simulink model "obs_com_filtro_2014"  (R2014b)
settings: Solver=ode45  SolverMode=SingleTasking  StartTime=0.0  StopTime=600  RelTol=1e-3
model workspace (MAT data in the model file):
  Td = 2
  std_dev = 0.08
values from neighbouring files (symbols this model uses):
  K = 0.002677    [run_and_calculate.m]
  T = 0.5    [run_and_calculate.m]
undefined symbols (not defined in the file): sigma_n
libraries: cstblocks x27
(part 1 of 2)
settings Model: CovMetricSettings=dwe  CovHtmlReporting=off  covSaveCumulativeToWorkspaceVar=off  CovSaveSingleToWorkspaceVar=off  CovExternalEMLEnable=on  CovSFcnEnable=on  Creator=Gabriel Vieira  LastModifiedBy=Gabriel Vieira
settings DataIOCC: LimitDataPoints=off  SaveFormat=StructureWithTime  ReturnWorkspaceOutputs=on
settings DebuggingCC: SolverPrmCheckMsg=none  FrameProcessingCompatibilityMsg=error  SFUnexpectedBacktrackingDiag=error  SFNoUnconditionalDefaultTransitionDiag=error
settings HardwareCC: ProdBitPerPointer=64  ProdLargestAtomicFloat=Float  ProdIntDivRoundTo=Zero  ProdEndianess=LittleEndian  ProdHWDeviceType=Specified
settings ModelReferenceCC: PropagateSignalLabelsOutOfModel=on
settings SFSimCC: SimUseLocalCustomCode=on
settings RTWCC: RTWUseLocalCustomCode=on
settings GRTTargetCC: TargetLangStandard=C99 (ISO)

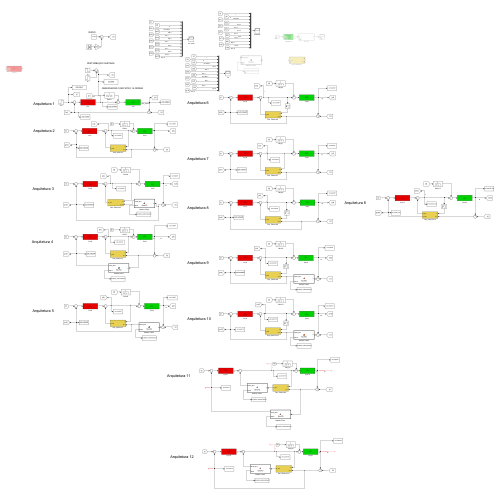
[thumbnail: Simulink's stored preview of the top-level diagram]
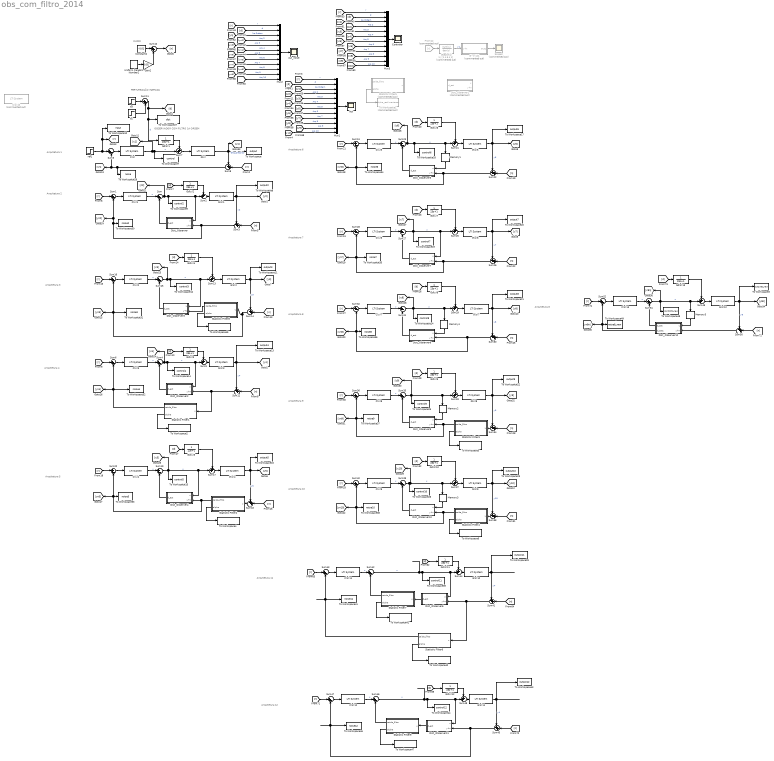
== system obs_com_filtro_2014 ==
  note: RUÍDO
  note: OBSERVADOR COM FILTRO 1A ORDEM
  note: PERTURBAÇÃO INJETADA
  note: Arquitetura 1
  note: Arquitetura 2
  note: Arquitetura 3
  note: Arquitetura 4
  note: Arquitetura 5
  note: Arquitetura 6
  note: Arquitetura 7
  note: Arquitetura 8
  note: Arquitetura 9
  note: Arquitetura 10
  note: Arquitetura 11
  note: Arquitetura 12
  note: Arquitetura 8
  C(s){,1..9,11..13} (13 alike) : cstblocks/LTI System  sys=C  IC=[]
  C(s)10 : cstblocks/LTI System  Commented=on  sys=C  IC=[]
  Constant2 : Constant  Value=-0.01
  Controler : Scope
      settings: TimeRange=auto  ShowLegends=on  MaxDataPoints=5000  SaveToWorkspace=off  YMin=-31.53639  YMax=49.84802  SampleTime=-1
  Dist_Observer : Subsystem  mask{Td=Td}
      mask prompts: Td "Filter time cte (Td)"
  Dist_Observer1 : Subsystem  Commented=on  mask{std_dev=std_dev}
      mask prompts: std_dev "Noise Std Deviation (std_dev)"
  Dist_Observer10 : Subsystem  mask{Td=Td, std_dev=std_dev}
      mask prompts: Td "Filter time cte (Td)"; std_dev "Noised Std Derivation"
  Dist_Observer11 : Subsystem  mask{Td=Td}
      mask prompts: Td "Filter time cte (Td)"
  Dist_Observer12 : Subsystem  mask{std_dev=std_dev}
      mask prompts: std_dev "Noised Std Derivation"
  Dist_Observer2 : Subsystem  mask{Td=Td}
      mask prompts: Td "Filter time cte (Td)"
  Dist_Observer3 : Subsystem  mask{Td=Td}
      mask prompts: Td "Filter time cte (Td)"
  Dist_Observer4 : Subsystem  mask{Td=Td}
      mask prompts: Td "Filter time cte (Td)"
  Dist_Observer5 : Subsystem  mask{Td=Td, std_dev=std_dev}
      mask prompts: Td "Filter time cte (Td)"; std_dev "Noised Std Derivation"
  Dist_Observer6 : Subsystem  mask{Td=Td}
      mask prompts: Td "Filter time cte (Td)"
  Dist_Observer7 : Subsystem  mask{Td=Td, std_dev=std_dev}
      mask prompts: Td "Filter time cte (Td)"; std_dev "Noised Std Derivation"
  Dist_Observer8 : Subsystem  mask{std_dev=std_dev}
      mask prompts: std_dev "Noised Std Derivation"
  Dist_Observer9 : Subsystem  mask{Td=Td, std_dev=std_dev}
      mask prompts: Td "Filter time cte (Td)"; std_dev "Noised Std Derivation"
  From12 : From  Commented=on  GotoTag=r
  G(s){,1..12} (13 alike) : cstblocks/LTI System  sys=Gs  IC=[]
  "G^{-1}1" : Subsystem  Commented=on
  Gain2 : Gain  Gain=0.02
  Gd(s){1..13} (13 alike) : TransferFcn  Numerator=1  Denominator=[23 1]
  Gteste(s) : TransferFcn  Commented=on  Numerator=1  Denominator=[1 4 6 4 1]
  Memory{1..5} (5 alike) : Memory
  Mux1 : Mux  Inputs=12
  Mux2 : Mux  Inputs=12
  Mux3 : Mux  Inputs=12
  Scope2 : Scope  Commented=on
  Statistic Filter1 : MATLAB Function  TreatAsAtomicUnit=on  mask{std_dev=sigma_n}
      mask prompts: std_dev "Noise Std Deviation (std_dev)"
      settings: PermitHierarchicalResolution=ParametersOnly
  Statistic Filter2 : MATLAB Function  TreatAsAtomicUnit=on  mask{std_dev=sigma_n}
      mask prompts: std_dev "Noise Std Deviation (std_dev)"
      settings: PermitHierarchicalResolution=ParametersOnly
  Statistic Filter3 : MATLAB Function  TreatAsAtomicUnit=on  mask{std_dev=sigma_n}
      mask prompts: std_dev "Noise Std Deviation (std_dev)"
      settings: PermitHierarchicalResolution=ParametersOnly
  Statistic Filter4 : MATLAB Function  TreatAsAtomicUnit=on  mask{std_dev=sigma_n}
      mask prompts: std_dev "Noise Std Deviation (std_dev)"
      settings: PermitHierarchicalResolution=ParametersOnly
  Statistic Filter5 : MATLAB Function  Commented=on  TreatAsAtomicUnit=on  mask{std_dev=0.5}
      mask prompts: std_dev "Noise Std Deviation (std_dev)"
      settings: PermitHierarchicalResolution=ParametersOnly
  Statistic Filter6 : MATLAB Function  TreatAsAtomicUnit=on  mask{std_dev=sigma_n}
      mask prompts: std_dev "Noise Std Deviation (std_dev)"
      settings: PermitHierarchicalResolution=ParametersOnly
  Statistic Filter7 : MATLAB Function  TreatAsAtomicUnit=on  mask{std_dev=sigma_n*2}
      mask prompts: std_dev "Noise Std Deviation (std_dev)"
      settings: PermitHierarchicalResolution=ParametersOnly
  Statistic Filter8 : MATLAB Function  TreatAsAtomicUnit=on  mask{std_dev=sigma_n}
      mask prompts: std_dev "Noise Std Deviation (std_dev)"
      settings: PermitHierarchicalResolution=ParametersOnly
  Statistic Filter9 : MATLAB Function  TreatAsAtomicUnit=on  mask{std_dev=sigma_n}
      mask prompts: std_dev "Noise Std Deviation (std_dev)"
      settings: PermitHierarchicalResolution=ParametersOnly
  Sum{,1,4..6,15..16,19..20,23..24,27..28,31..32,35..36,39..40,42..43,46..47,51..52} (25 alike) : Sum  Inputs=|+-
  Sum10 : Sum  Inputs=|++
  Sum11 : Sum  Inputs=|++
  Sum{2..3,7..9,12..14,17..18,21..22,25..26,29..30,33..34,37..38,41,44..45,48..50} (26 alike) : Sum  Inputs=++|
  To Workspace : ToWorkspace  VariableName=output  SaveFormat=Timeseries  SampleTime=-1
  To Workspace1 : ToWorkspace  Commented=on  VariableName=alpha_realimentacao  SaveFormat=Timeseries  SampleTime=-1
  To Workspace10 : ToWorkspace  VariableName=input  SaveFormat=Timeseries  SampleTime=-1
  To Workspace11 : ToWorkspace  VariableName=output3  SaveFormat=Timeseries  SampleTime=-1
  To Workspace12 : ToWorkspace  VariableName=control3  SaveFormat=Timeseries  SampleTime=-1
  To Workspace13 : ToWorkspace  VariableName=output4  SaveFormat=Timeseries  SampleTime=-1
  To Workspace14 : ToWorkspace  VariableName=control4  SaveFormat=Timeseries  SampleTime=-1
  To Workspace15 : ToWorkspace  VariableName=control5  SaveFormat=Timeseries  SampleTime=-1
  To Workspace16 : ToWorkspace  VariableName=output5  SaveFormat=Timeseries  SampleTime=-1
  To Workspace17 : ToWorkspace  VariableName=output6  SaveFormat=Timeseries  SampleTime=-1
  To Workspace18 : ToWorkspace  VariableName=control6  SaveFormat=Timeseries  SampleTime=-1
  To Workspace19 : ToWorkspace  VariableName=control7  SaveFormat=Timeseries  SampleTime=-1
  To Workspace2 : ToWorkspace  VariableName=alpha_realimentacao1  SaveFormat=Timeseries  SampleTime=-1
  To Workspace20 : ToWorkspace  VariableName=output7  SaveFormat=Timeseries  SampleTime=-1
  To Workspace21 : ToWorkspace  VariableName=output8  SaveFormat=Timeseries  SampleTime=-1
  To Workspace22 : ToWorkspace  VariableName=output9  SaveFormat=Timeseries  SampleTime=-1
  To Workspace23 : ToWorkspace  VariableName=output10  SaveFormat=Timeseries  SampleTime=-1
  To Workspace24 : ToWorkspace  VariableName=control8  SaveFormat=Timeseries  SampleTime=-1
  To Workspace25 : ToWorkspace  VariableName=control9  SaveFormat=Timeseries  SampleTime=-1
  To Workspace26 : ToWorkspace  VariableName=control10  SaveFormat=Timeseries  SampleTime=-1
  To Workspace27 : ToWorkspace  VariableName=dist  SaveFormat=Timeseries  SampleTime=-1
  To Workspace28 : ToWorkspace  VariableName=noise  SaveFormat=Timeseries  SampleTime=-1
  To Workspace29 : ToWorkspace  VariableName=output11  SaveFormat=Timeseries  SampleTime=-1
  To Workspace3 : ToWorkspace  VariableName=output8_new  SaveFormat=Timeseries  SampleTime=-1
  To Workspace30 : ToWorkspace  VariableName=noise2  SaveFormat=Timeseries  SampleTime=-1
  To Workspace31 : ToWorkspace  VariableName=noise3  SaveFormat=Timeseries  SampleTime=-1
  To Workspace32 : ToWorkspace  VariableName=noise4  SaveFormat=Timeseries  SampleTime=-1
  To Workspace33 : ToWorkspace  VariableName=noise5  SaveFormat=Timeseries  SampleTime=-1
  To Workspace34 : ToWorkspace  VariableName=noise6  SaveFormat=Timeseries  SampleTime=-1
  To Workspace35 : ToWorkspace  VariableName=noise7  SaveFormat=Timeseries  SampleTime=-1
  To Workspace36 : ToWorkspace  VariableName=noise8  SaveFormat=Timeseries  SampleTime=-1
  To Workspace37 : ToWorkspace  VariableName=noise9  SaveFormat=Timeseries  SampleTime=-1
  To Workspace38 : ToWorkspace  VariableName=noise10  SaveFormat=Timeseries  SampleTime=-1
  To Workspace39 : ToWorkspace  VariableName=control11  SaveFormat=Timeseries  SampleTime=-1
  To Workspace4 : ToWorkspace  VariableName=alpha_realimentacao3  SaveFormat=Timeseries  SampleTime=-1
  To Workspace40 : ToWorkspace  VariableName=alpha_realimentacao11  SaveFormat=Timeseries  SampleTime=-1
  To Workspace41 : ToWorkspace  VariableName=noise11  SaveFormat=Timeseries  SampleTime=-1
  To Workspace42 : ToWorkspace  VariableName=alpha_realimentacao8  SaveFormat=Timeseries  SampleTime=-1
  To Workspace43 : ToWorkspace  VariableName=output12  SaveFormat=Timeseries  SampleTime=-1
  To Workspace44 : ToWorkspace  VariableName=control12  SaveFormat=Timeseries  SampleTime=-1
  To Workspace45 : ToWorkspace  VariableName=alpha_realimentacao9  SaveFormat=Timeseries  SampleTime=-1
  To Workspace46 : ToWorkspace  VariableName=noise12  SaveFormat=Timeseries  SampleTime=-1
  To Workspace47 : ToWorkspace  VariableName=alpha_realimentacao12  SaveFormat=Timeseries  SampleTime=-1
  To Workspace48 : ToWorkspace  VariableName=control8_new  SaveFormat=Timeseries  SampleTime=-1
  To Workspace49 : ToWorkspace  VariableName=noise8_new  SaveFormat=Timeseries  SampleTime=-1
  To Workspace5 : ToWorkspace  VariableName=alpha_realimentacao4  SaveFormat=Timeseries  SampleTime=-1
  To Workspace6 : ToWorkspace  VariableName=alpha_realimentacao6  SaveFormat=Timeseries  SampleTime=-1
  To Workspace7 : ToWorkspace  VariableName=control  SaveFormat=Timeseries  SampleTime=-1
  To Workspace8 : ToWorkspace  VariableName=output2  SaveFormat=Timeseries  SampleTime=-1
  To Workspace9 : ToWorkspace  VariableName=control2  SaveFormat=Timeseries  SampleTime=-1
  Uniform Random Number2 : UniformRandomNumber  SampleTime=0.01
  d2 : Step  Time=150  SampleTime=0
  d3 : Step  Time=200  After=-1  SampleTime=0
  out : Scope
  out_noise : Scope
  ref1 : Step  Time=50  SampleTime=0
  wires:
  Sum10/1 -> [n]
  Constant2/1 -> Sum10/1
  Sum5/1 -> C(s)/1
  d2/1 -> Sum11/2
  C(s)/1 -> [c1], To Workspace7/1, Sum7/2  "u"
  Gain2/1 -> Sum10/2
  ref1/1 -> To Workspace10/1, [r], Sum5/1
  Uniform Random Number2/1 -> Gain2/1
  Mux1/1 -> out/1
  Sum7/1 -> G(s)/1
  Sum11/1 -> [d], To Workspace27/1, Gd(s)1/1  "d"
  Gd(s)1/1 -> Sum7/1
  [n] -> Sum8/2
  d3/1 -> Sum11/1
  G(s)/1 -> [y1], Sum8/1, To Workspace/1  "Obs_Classico"
  Sum8/1 -> To Workspace28/1, [yn], Sum5/2
  [n] -> Sum3/2
  Gd(s)2/1 -> Sum2/1
  Sum2/1 -> G(s)1/1
  Sum1/1 -> C(s)1/1
  [r] -> Sum1/1
  [d] -> Gd(s)2/1
  C(s)1/1 -> Sum/1  "u"
  Sum3/1 -> Dist_Observer/2(y+n), To Workspace30/1, [yn2], Sum1/2
  Dist_Observer/1(d_est) -> Sum/2
  G(s)1/1 -> To Workspace8/1, [y2], Sum3/1  "y2"
  Statistic Filter5/2(alpha) -> To Workspace1/1
  Sum9/1 -> G(s)3/1
  Gd(s)3/1 -> Sum9/1
  G(s)3/1 -> To Workspace13/1, [y4], Sum12/1  "y4"
  [r] -> Sum6/1
  [d] -> Gd(s)3/1
  C(s)3/1 -> Sum4/1  "u"
  Dist_Observer2/1(d_est) -> Sum4/2
  Sum6/1 -> C(s)3/1
  [n] -> Sum12/2
  Sum12/1 -> Statistic Filter1/1(u), Dist_Observer2/2(y+n)
  Statistic Filter1/2(alpha) -> To Workspace2/1
  Gteste(s)/1 -> "G^{-1}1"/1(y+n)  "y1"
  From12/1 -> Gteste(s)/1
  "G^{-1}1"/1(Out1) -> Scope2/1
  [d] -> Gd(s)4/1
  Sum13/1 -> G(s)2/1
  Gd(s)4/1 -> Sum13/1
  [n] -> Sum14/2
  G(s)2/1 -> Sum14/1, To Workspace11/1, [y3]  "y3"
  Sum16/1 -> C(s)2/1
  C(s)2/1 -> Sum15/1  "u"
  [r] -> Sum16/1
  Dist_Observer4/1(d_est) -> Sum19/2
  [r] -> Sum20/1
  Sum17/1 -> G(s)4/1
  Sum18/1 -> Statistic Filter2/1(u)
  Statistic Filter2/2(alpha) -> To Workspace4/1
  G(s)4/1 -> To Workspace16/1, [y5], Sum18/1  "y5"
  [d] -> Gd(s)5/1
  Sum20/1 -> C(s)4/1
  C(s)4/1 -> Sum19/1  "u"
  Gd(s)5/1 -> Sum17/1
  [n] -> Sum18/2
  [n] -> Sum22/2
  Gd(s)6/1 -> Sum21/1
  Sum24/1 -> C(s)5/1
  [d] -> Gd(s)6/1
  C(s)5/1 -> Sum23/1  "u"
  G(s)5/1 -> To Workspace17/1, [y6], Sum22/1  "y6"
  Dist_Observer5/1(d_est) -> Sum23/2
  Sum21/1 -> G(s)5/1
  [r] -> Sum24/1
  Gd(s)7/1 -> Sum25/1
  [n] -> Sum26/2
  G(s)6/1 -> To Workspace20/1, [y7], Sum26/1  "y7"
  Sum28/1 -> C(s)6/1
  C(s)6/1 -> Sum27/1  "u"
  [r] -> Sum28/1
  Dist_Observer7/1(d_est) -> Sum27/2
  [d] -> Gd(s)7/1
  Sum25/1 -> G(s)6/1
  Gd(s)8/1 -> Sum29/1
  Dist_Observer8/1(d_est) -> Sum31/2
  [r] -> Sum32/1
  C(s)7/1 -> Sum31/1  "u"
  Sum32/1 -> C(s)7/1
  [n] -> Sum30/2
  G(s)7/1 -> To Workspace21/1, [y8], Sum30/1  "y8"
  Sum29/1 -> G(s)7/1
  Sum38/1 -> Statistic Filter4/1(u)
  Statistic Filter4/2(alpha) -> To Workspace6/1
  Gd(s)10/1 -> Sum37/1
  Dist_Observer10/1(d_est) -> Sum39/2
  G(s)9/1 -> To Workspace23/1, [y10], Sum38/1  "y10"
  [n] -> Sum38/2
  Sum34/1 -> Statistic Filter3/1(u)
  Sum40/1 -> C(s)9/1
  C(s)9/1 -> Sum39/1  "u"
  Statistic Filter3/2(alpha) -> To Workspace5/1
  Gd(s)9/1 -> Sum33/1
  Sum35/1 -> [c9], To Workspace25/1, Memory2/1, Sum33/2
  [n] -> Sum34/2
  G(s)8/1 -> [y9], To Workspace22/1, Sum34/1  "y9"
  [r] -> Sum36/1
  [r] -> Sum40/1
  Dist_Observer9/1(d_est) -> Sum35/2
  [d] -> Gd(s)9/1
  Sum33/1 -> G(s)8/1
  Sum37/1 -> G(s)9/1
  Sum36/1 -> C(s)8/1
  C(s)8/1 -> Sum35/1  "u"
  [d] -> Gd(s)10/1
  [r] -> Mux2/1  "r"
  [d] -> Mux2/2  "d"
  Mux2/1 -> out_noise/1
  [yn] -> Mux2/3  "1a Ordem"
  Sum14/1 -> Statistic Filter8/1(u), To Workspace31/1, [yn3], Sum16/2
  Statistic Filter1/1(saida_filtro) -> Sum6/2, To Workspace32/1, [yn4]
  Statistic Filter2/1(saida_filtro) -> Dist_Observer4/2(y+n), To Workspace33/1, [yn5], Sum20/2
  Sum22/1 -> Dist_Observer5/2(y+n), To Workspace34/1, [yn6], Sum24/2
  Sum26/1 -> Dist_Observer7/2(y+n), To Workspace35/1, [yn7], Sum28/2
  Statistic Filter3/1(saida_filtro) -> Dist_Observer9/2(y+n), To Workspace37/1, [yn9], Sum36/2
  Statistic Filter4/1(saida_filtro) -> Dist_Observer10/2(y+n), To Workspace38/1, [yn10], Sum40/2
  Memory2/1 -> Dist_Observer9/1(u)
  Memory3/1 -> Dist_Observer10/1(u)
  [yn8] -> Mux2/10  "Arq 8"
  [yn7] -> Mux2/9  "Arq 7"
  [yn6] -> Mux2/8  "Arq 6"
  [yn5] -> Mux2/7  "Arq 5"
  [yn4] -> Mux2/6  "Arq 4"
  [yn3] -> Mux2/5  "Arq 3"
  [yn2] -> Mux2/4  "Arq 2"
  Mux3/1 -> Controler/1
  Sum15/1 -> [c3], To Workspace12/1, Dist_Observer3/1(u), Sum13/2  "u"
  Sum4/1 -> [c4], To Workspace14/1, Dist_Observer2/1(u), Sum9/2  "u"
  Sum19/1 -> [c5], To Workspace15/1, Dist_Observer4/1(u), Sum17/2  "u"
  Sum23/1 -> [c6], To Workspace18/1, Memory1/1, Sum21/2  "u"
  Sum27/1 -> [c7], To Workspace19/1, Dist_Observer7/1(u), Sum25/2  "u"
  Sum31/1 -> [c8], Memory4/1, Sum29/2, To Workspace24/1  "u"
  Sum39/1 -> To Workspace26/1, [c10], Memory3/1, Sum37/2  "u"
  [r] -> Mux3/1  "r"
  [d] -> Mux3/2  "d"
  Sum/1 -> [c2], To Workspace9/1, Dist_Observer/1(u), Sum2/2
  Statistic Filter8/1(saida_filtro) -> Dist_Observer3/2(y+n)
  Dist_Observer3/1(d_est) -> Sum15/2
  [y2] -> Mux1/4  "Arq 2"
  [y7] -> Mux1/9  "Arq 7"
  [y6] -> Mux1/8  "Arq 6"
  [y4] -> Mux1/6  "Arq 4"
  [y8] -> Mux1/10  "Arq 8"
  [y3] -> Mux1/5  "Arq 3"
  [y1] -> Mux1/3  "1a Ordem"
  [d] -> Mux1/2  "d"
  [r] -> Mux1/1  "r"
  [y5] -> Mux1/7  "Arq 5"
  [c2] -> Mux3/4  "Arq 2"
  [c5] -> Mux3/7  "Arq 5"
  [c7] -> Mux3/9  "Arq 7"
  [c6] -> Mux3/8  "Arq 6"
  [c4] -> Mux3/6  "Arq 4"
  [c8] -> Mux3/10  "Arq 8"
  [c1] -> Mux3/3  "1a Ordem"
  [c3] -> Mux3/5  "Arq 3"
  [yn10] -> Mux2/12  "Arq 10"
  [c10] -> Mux3/12  "Arq 10"
  [y10] -> Mux1/12  "Arq 10"
  [yn9] -> Mux2/11  "Arq 9"
  [c9] -> Mux3/11  "Arq 9"
  [y9] -> Mux1/11  "Arq 9"
  [d] -> Gd(s)8/1
  Statistic Filter6/1(saida_filtro) -> Sum43/2, To Workspace41/1
  Sum42/1 -> To Workspace39/1, Dist_Observer6/1(u), Sum44/2  "u"
  Gd(s)11/1 -> Sum44/1
  Sum41/1 -> Statistic Filter6/1(u), Dist_Observer6/2(y+n)
  Sum44/1 -> G(s)10/1
  G(s)10/1 -> To Workspace29/1, Sum41/1  "y4"
  [d] -> Gd(s)11/1
  C(s)11/1 -> Sum42/1  "u"
  [n] -> Sum41/2
  Sum43/1 -> C(s)11/1
  Statistic Filter6/2(alpha) -> To Workspace40/1
  [r] -> Sum43/1
  Dist_Observer6/1(d_est) -> Statistic Filter7/1(u)
  Statistic Filter7/2(alpha) -> To Workspace42/1
  Statistic Filter7/1(saida_filtro) -> Sum42/2
  Dist_Observer11/1(d_est) -> Statistic Filter9/1(u)
  Statistic Filter9/2(alpha) -> To Workspace47/1
  Sum47/1 -> C(s)12/1
  [n] -> Sum45/2
  [r] -> Sum47/1
  [d] -> Gd(s)12/1
  C(s)12/1 -> Sum46/1  "u"
  Sum48/1 -> G(s)11/1
  G(s)11/1 -> To Workspace43/1, Sum45/1  "y4"
  Gd(s)12/1 -> Sum48/1
  Sum45/1 -> To Workspace46/1, Sum47/2, Dist_Observer11/2(y+n)
  Sum46/1 -> To Workspace44/1, Dist_Observer11/1(u), Sum48/2  "u"
  Statistic Filter9/1(saida_filtro) -> Sum46/2
  Statistic Filter8/2(alpha) -> To Workspace45/1
  Sum30/1 -> Sum32/2, [yn8], To Workspace36/1, Dist_Observer8/2(y+n)
  Dist_Observer12/2(d_est1) -> [yn8n], To Workspace49/1, Sum52/2
  [r] -> Sum52/1
  Dist_Observer12/1(d_est) -> Sum51/2
  [d] -> Gd(s)13/1
  Sum52/1 -> C(s)13/1
  Sum50/1 -> Dist_Observer12/2(y+n)
  Sum49/1 -> G(s)12/1
  G(s)12/1 -> To Workspace3/1, [y8n], Sum50/1  "y8"
  Sum51/1 -> [c8n], Memory5/1, Sum49/2, To Workspace48/1  "u"
  [n] -> Sum50/2
  C(s)13/1 -> Sum51/1  "u"
  Gd(s)13/1 -> Sum49/1
  Memory1/1 -> Dist_Observer5/1(u)
  Memory4/1 -> Dist_Observer8/1(u)
  Memory5/1 -> Dist_Observer12/1(u)

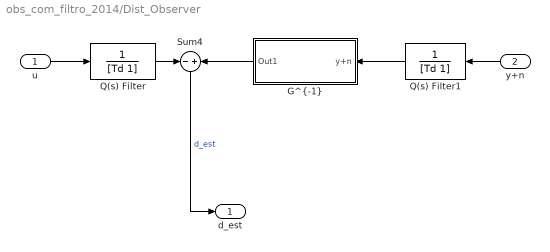
== system obs_com_filtro_2014/Dist_Observer ==
  u : Inport
  y+n : Inport  Port=2
  "G^{-1}" : Subsystem
  Q(s) Filter : TransferFcn  Denominator=[Td 1]
  Q(s) Filter1 : TransferFcn  Denominator=[Td 1]
  Sum4 : Sum  Inputs=-|+
  d_est : Outport
  wires:
  Q(s) Filter/1 -> Sum4/1
  Sum4/1 -> d_est/1  "d_est"
  u/1 -> Q(s) Filter/1
  "G^{-1}"/1(Out1) -> Sum4/2
  Q(s) Filter1/1 -> "G^{-1}"/1(y+n)
  y+n/1 -> Q(s) Filter1/1

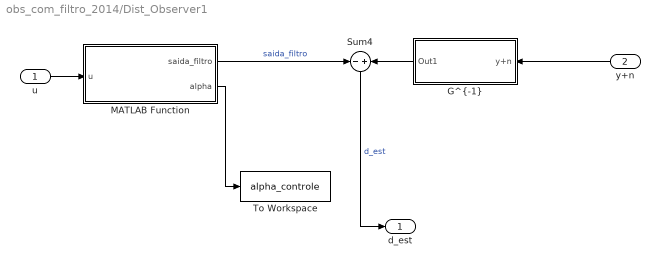
== system obs_com_filtro_2014/Dist_Observer1 ==
  u : Inport
  y+n : Inport  Port=2
  "G^{-1}" : Subsystem
  MATLAB Function : MATLAB Function  TreatAsAtomicUnit=on
      settings: PermitHierarchicalResolution=ParametersOnly
  Sum4 : Sum  Inputs=-|+
  To Workspace : ToWorkspace  VariableName=alpha_controle  SaveFormat=Timeseries  SampleTime=-1
  d_est : Outport
  wires:
  MATLAB Function/1(saida_filtro) -> Sum4/1  "saida_filtro"
  Sum4/1 -> d_est/1  "d_est"
  u/1 -> MATLAB Function/1(u)
  "G^{-1}"/1(Out1) -> Sum4/2
  MATLAB Function/2(alpha) -> To Workspace/1
  y+n/1 -> "G^{-1}"/1(y+n)

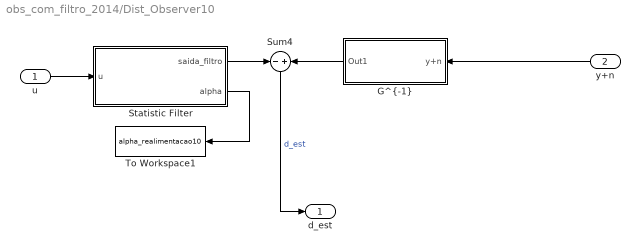
== system obs_com_filtro_2014/Dist_Observer10 ==
  u : Inport
  y+n : Inport  Port=2
  "G^{-1}" : Subsystem
  Statistic Filter : MATLAB Function  TreatAsAtomicUnit=on  mask{std_dev=sigma_n}
      mask prompts: std_dev "Noise Std Deviation (std_dev)"
      settings: PermitHierarchicalResolution=ParametersOnly
  Sum4 : Sum  Inputs=-|+
  To Workspace1 : ToWorkspace  VariableName=alpha_realimentacao10  SaveFormat=Timeseries  SampleTime=-1
  d_est : Outport
  wires:
  Statistic Filter/1(saida_filtro) -> Sum4/1
  Sum4/1 -> d_est/1  "d_est"
  u/1 -> Statistic Filter/1(u)
  "G^{-1}"/1(Out1) -> Sum4/2
  y+n/1 -> "G^{-1}"/1(y+n)
  Statistic Filter/2(alpha) -> To Workspace1/1

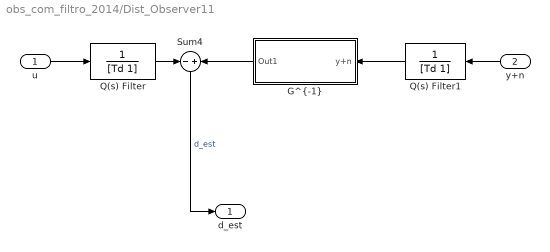
== system obs_com_filtro_2014/Dist_Observer11 ==
  u : Inport
  y+n : Inport  Port=2
  "G^{-1}" : Subsystem
  Q(s) Filter : TransferFcn  Denominator=[Td 1]
  Q(s) Filter1 : TransferFcn  Denominator=[Td 1]
  Sum4 : Sum  Inputs=-|+
  d_est : Outport
  wires:
  Q(s) Filter/1 -> Sum4/1
  Sum4/1 -> d_est/1  "d_est"
  u/1 -> Q(s) Filter/1
  "G^{-1}"/1(Out1) -> Sum4/2
  Q(s) Filter1/1 -> "G^{-1}"/1(y+n)
  y+n/1 -> Q(s) Filter1/1

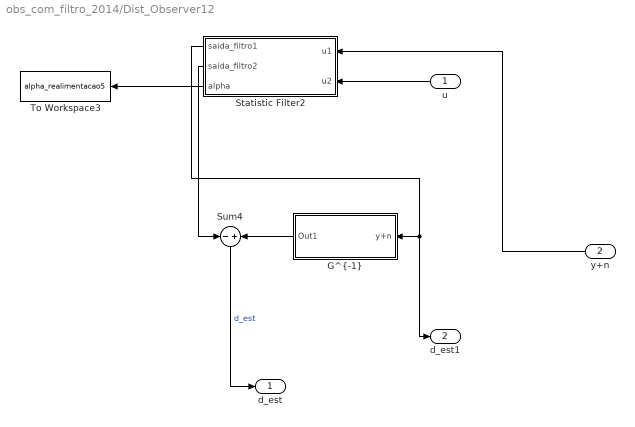
== system obs_com_filtro_2014/Dist_Observer12 ==
  u : Inport
  y+n : Inport  Port=2
  "G^{-1}" : Subsystem
  Statistic Filter2 : MATLAB Function  TreatAsAtomicUnit=on  mask{std_dev=sigma_n*2, alpha_max=0.008}
      mask prompts: std_dev "Noise Std Deviation (std_dev)"; alpha_max "Maximum value of alpha"
      settings: PermitHierarchicalResolution=ParametersOnly
  Sum4 : Sum  Inputs=-|+
  To Workspace3 : ToWorkspace  VariableName=alpha_realimentacao5  SaveFormat=Timeseries  SampleTime=-1
  d_est : Outport
  d_est1 : Outport  Port=2
  wires:
  Sum4/1 -> d_est/1  "d_est"
  "G^{-1}"/1(Out1) -> Sum4/2
  Statistic Filter2/2(saida_filtro2) -> Sum4/1
  u/1 -> Statistic Filter2/2(u2)
  Statistic Filter2/1(saida_filtro1) -> d_est1/1, "G^{-1}"/1(y+n)
  y+n/1 -> Statistic Filter2/1(u1)
  Statistic Filter2/3(alpha) -> To Workspace3/1

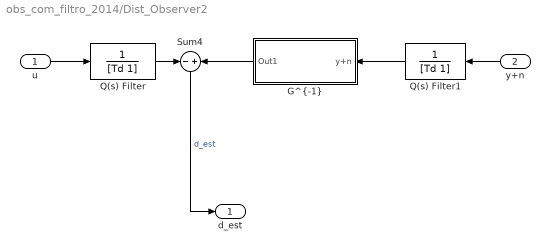
== system obs_com_filtro_2014/Dist_Observer2 ==
  u : Inport
  y+n : Inport  Port=2
  "G^{-1}" : Subsystem
  Q(s) Filter : TransferFcn  Denominator=[Td 1]
  Q(s) Filter1 : TransferFcn  Denominator=[Td 1]
  Sum4 : Sum  Inputs=-|+
  d_est : Outport
  wires:
  Q(s) Filter/1 -> Sum4/1
  Sum4/1 -> d_est/1  "d_est"
  u/1 -> Q(s) Filter/1
  "G^{-1}"/1(Out1) -> Sum4/2
  Q(s) Filter1/1 -> "G^{-1}"/1(y+n)
  y+n/1 -> Q(s) Filter1/1

== system obs_com_filtro_2014/Dist_Observer3 ==
  u : Inport
  y+n : Inport  Port=2
  "G^{-1}" : Subsystem
  Q(s) Filter : TransferFcn  Denominator=[Td 1]
  Q(s) Filter1 : TransferFcn  Denominator=[Td 1]
  Sum4 : Sum  Inputs=-|+
  d_est : Outport
  wires:
  Q(s) Filter/1 -> Sum4/1
  Sum4/1 -> d_est/1  "d_est"
  u/1 -> Q(s) Filter/1
  "G^{-1}"/1(Out1) -> Sum4/2
  Q(s) Filter1/1 -> "G^{-1}"/1(y+n)
  y+n/1 -> Q(s) Filter1/1

== system obs_com_filtro_2014/Dist_Observer4 ==
  u : Inport
  y+n : Inport  Port=2
  "G^{-1}" : Subsystem
  Q(s) Filter : TransferFcn  Denominator=[Td 1]
  Q(s) Filter1 : TransferFcn  Denominator=[Td 1]
  Sum4 : Sum  Inputs=-|+
  d_est : Outport
  wires:
  Q(s) Filter/1 -> Sum4/1
  Sum4/1 -> d_est/1  "d_est"
  u/1 -> Q(s) Filter/1
  "G^{-1}"/1(Out1) -> Sum4/2
  Q(s) Filter1/1 -> "G^{-1}"/1(y+n)
  y+n/1 -> Q(s) Filter1/1

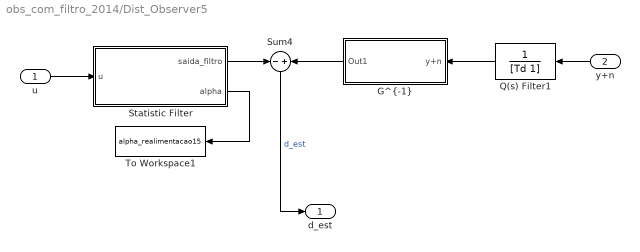
== system obs_com_filtro_2014/Dist_Observer5 ==
  u : Inport
  y+n : Inport  Port=2
  "G^{-1}" : Subsystem
  Q(s) Filter1 : TransferFcn  Denominator=[Td 1]
  Statistic Filter : MATLAB Function  TreatAsAtomicUnit=on  mask{std_dev=0.5}
      mask prompts: std_dev "Noise Std Deviation (std_dev)"
      settings: PermitHierarchicalResolution=ParametersOnly
  Sum4 : Sum  Inputs=-|+
  To Workspace1 : ToWorkspace  VariableName=alpha_realimentacao15  SaveFormat=Timeseries  SampleTime=-1
  d_est : Outport
  wires:
  Statistic Filter/1(saida_filtro) -> Sum4/1
  Sum4/1 -> d_est/1  "d_est"
  u/1 -> Statistic Filter/1(u)
  "G^{-1}"/1(Out1) -> Sum4/2
  Q(s) Filter1/1 -> "G^{-1}"/1(y+n)
  y+n/1 -> Q(s) Filter1/1
  Statistic Filter/2(alpha) -> To Workspace1/1

== system obs_com_filtro_2014/Dist_Observer6 ==
  u : Inport
  y+n : Inport  Port=2
  "G^{-1}" : Subsystem
  Q(s) Filter : TransferFcn  Denominator=[Td 1]
  Q(s) Filter1 : TransferFcn  Denominator=[Td 1]
  Sum4 : Sum  Inputs=-|+
  d_est : Outport
  wires:
  Q(s) Filter/1 -> Sum4/1
  Sum4/1 -> d_est/1  "d_est"
  u/1 -> Q(s) Filter/1
  "G^{-1}"/1(Out1) -> Sum4/2
  Q(s) Filter1/1 -> "G^{-1}"/1(y+n)
  y+n/1 -> Q(s) Filter1/1

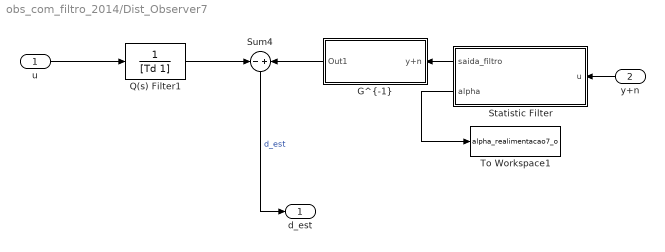
== system obs_com_filtro_2014/Dist_Observer7 ==
  u : Inport
  y+n : Inport  Port=2
  "G^{-1}" : Subsystem
  Q(s) Filter1 : TransferFcn  Denominator=[Td 1]
  Statistic Filter : MATLAB Function  TreatAsAtomicUnit=on  mask{std_dev=sigma_n}
      mask prompts: std_dev "Noise Std Deviation (std_dev)"
      settings: PermitHierarchicalResolution=ParametersOnly
  Sum4 : Sum  Inputs=-|+
  To Workspace1 : ToWorkspace  VariableName=alpha_realimentacao7_o  SaveFormat=Timeseries  SampleTime=-1
  d_est : Outport
  wires:
  Sum4/1 -> d_est/1  "d_est"
  "G^{-1}"/1(Out1) -> Sum4/2
  Statistic Filter/2(alpha) -> To Workspace1/1
  Q(s) Filter1/1 -> Sum4/1
  u/1 -> Q(s) Filter1/1
  Statistic Filter/1(saida_filtro) -> "G^{-1}"/1(y+n)
  y+n/1 -> Statistic Filter/1(u)

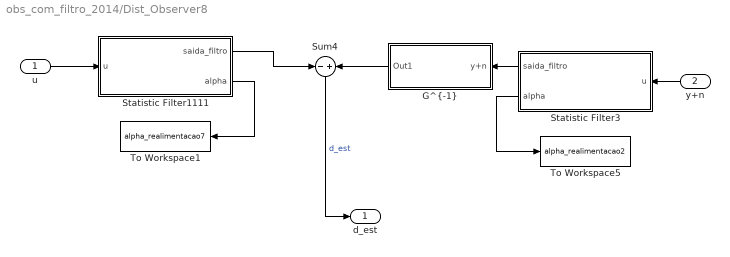
== system obs_com_filtro_2014/Dist_Observer8 ==
  u : Inport
  y+n : Inport  Port=2
  "G^{-1}" : Subsystem
  Statistic Filter1111 : MATLAB Function  TreatAsAtomicUnit=on  mask{std_dev=sigma_n}
      mask prompts: std_dev "Noise Std Deviation (std_dev)"
      settings: PermitHierarchicalResolution=ParametersOnly
  Statistic Filter3 : MATLAB Function  TreatAsAtomicUnit=on  mask{std_dev=sigma_n}
      mask prompts: std_dev "Noise Std Deviation (std_dev)"
      settings: PermitHierarchicalResolution=ParametersOnly
  Sum4 : Sum  Inputs=-|+
  To Workspace1 : ToWorkspace  VariableName=alpha_realimentacao7  SaveFormat=Timeseries  SampleTime=-1
  To Workspace5 : ToWorkspace  VariableName=alpha_realimentacao2  SaveFormat=Timeseries  SampleTime=-1
  d_est : Outport
  wires:
  Sum4/1 -> d_est/1  "d_est"
  "G^{-1}"/1(Out1) -> Sum4/2
  y+n/1 -> Statistic Filter3/1(u)
  Statistic Filter3/1(saida_filtro) -> "G^{-1}"/1(y+n)
  Statistic Filter3/2(alpha) -> To Workspace5/1
  u/1 -> Statistic Filter1111/1(u)
  Statistic Filter1111/1(saida_filtro) -> Sum4/1
  Statistic Filter1111/2(alpha) -> To Workspace1/1

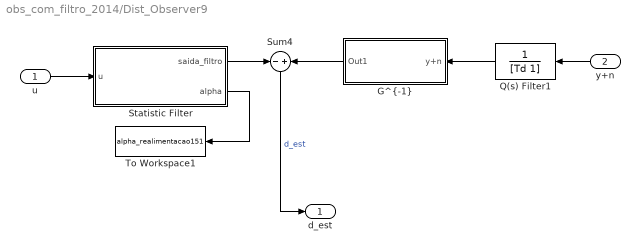
== system obs_com_filtro_2014/Dist_Observer9 ==
  u : Inport
  y+n : Inport  Port=2
  "G^{-1}" : Subsystem
  Q(s) Filter1 : TransferFcn  Denominator=[Td 1]
  Statistic Filter : MATLAB Function  TreatAsAtomicUnit=on  mask{std_dev=sigma_n}
      mask prompts: std_dev "Noise Std Deviation (std_dev)"
      settings: PermitHierarchicalResolution=ParametersOnly
  Sum4 : Sum  Inputs=-|+
  To Workspace1 : ToWorkspace  VariableName=alpha_realimentacao151  SaveFormat=Timeseries  SampleTime=-1
  d_est : Outport
  wires:
  Statistic Filter/1(saida_filtro) -> Sum4/1
  Sum4/1 -> d_est/1  "d_est"
  u/1 -> Statistic Filter/1(u)
  "G^{-1}"/1(Out1) -> Sum4/2
  Q(s) Filter1/1 -> "G^{-1}"/1(y+n)
  y+n/1 -> Q(s) Filter1/1
  Statistic Filter/2(alpha) -> To Workspace1/1

== system obs_com_filtro_2014/G^{-1}1 ==
  y+n : Inport
  Derivative : Derivative  CoefficientInTFapproximation=1e-6
  Sum : Sum  Inputs=|++
  Out1 : Outport
  wires:
  Derivative/1 -> Sum/2
  Sum/1 -> Out1/1
  y+n/1 -> Derivative/1, Sum/1

== system obs_com_filtro_2014/Dist_Observer/G^{-1} ==
  y+n : Inport
  Derivative : Derivative  CoefficientInTFapproximation=1e-6
  Gain : Gain  Gain=1/K
  Gain1 : Gain  Gain=T
  Sum : Sum  Inputs=|++
  Out1 : Outport
  wires:
  Gain/1 -> Gain1/1, Sum/1
  Sum/1 -> Out1/1
  Derivative/1 -> Sum/2
  Gain1/1 -> Derivative/1
  y+n/1 -> Gain/1

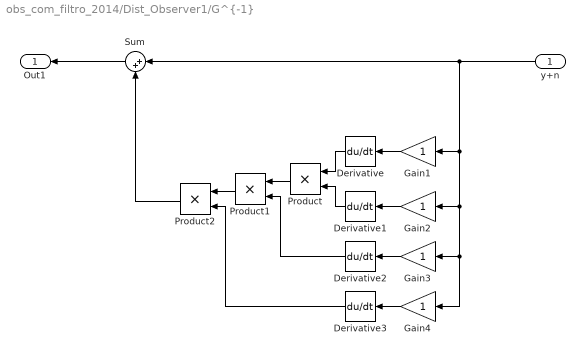
== system obs_com_filtro_2014/Dist_Observer1/G^{-1} ==
  y+n : Inport
  Derivative{,1..3} (4 alike) : Derivative  CoefficientInTFapproximation=1e-6
  Gain{1..4} (4 alike) : Gain
  Product : Product
  Product1 : Product
  Product2 : Product
  Sum : Sum  Inputs=|++
  Out1 : Outport
  wires:
  Sum/1 -> Out1/1
  Gain1/1 -> Derivative/1
  Derivative/1 -> Product/1
  Gain2/1 -> Derivative1/1
  Derivative1/1 -> Product/2
  Gain3/1 -> Derivative2/1
  y+n/1 -> Sum/1, Gain4/1, Gain3/1, Gain2/1, Gain1/1
  Gain4/1 -> Derivative3/1
  Product/1 -> Product1/1
  Derivative2/1 -> Product1/2
  Product1/1 -> Product2/1
  Derivative3/1 -> Product2/2
  Product2/1 -> Sum/2

== system obs_com_filtro_2014/Dist_Observer10/G^{-1} ==
  y+n : Inport
  Derivative : Derivative  CoefficientInTFapproximation=1e-6
  Gain : Gain  Gain=1/K
  Gain1 : Gain  Gain=T
  Sum : Sum  Inputs=|++
  Out1 : Outport
  wires:
  Gain/1 -> Gain1/1, Sum/1
  Sum/1 -> Out1/1
  Derivative/1 -> Sum/2
  Gain1/1 -> Derivative/1
  y+n/1 -> Gain/1

== system obs_com_filtro_2014/Dist_Observer11/G^{-1} ==
  y+n : Inport
  Derivative : Derivative  CoefficientInTFapproximation=1e-6
  Gain : Gain  Gain=1/K
  Gain1 : Gain  Gain=T
  Sum : Sum  Inputs=|++
  Out1 : Outport
  wires:
  Gain/1 -> Gain1/1, Sum/1
  Sum/1 -> Out1/1
  Derivative/1 -> Sum/2
  Gain1/1 -> Derivative/1
  y+n/1 -> Gain/1

== system obs_com_filtro_2014/Dist_Observer12/G^{-1} ==
  y+n : Inport
  Derivative : Derivative  CoefficientInTFapproximation=1e-6
  Gain : Gain  Gain=1/K
  Gain1 : Gain  Gain=T
  Sum : Sum  Inputs=|++
  Out1 : Outport
  wires:
  Gain/1 -> Gain1/1, Sum/1
  Sum/1 -> Out1/1
  Derivative/1 -> Sum/2
  Gain1/1 -> Derivative/1
  y+n/1 -> Gain/1

== system obs_com_filtro_2014/Dist_Observer2/G^{-1} ==
  y+n : Inport
  Derivative : Derivative  CoefficientInTFapproximation=1e-6
  Gain : Gain  Gain=1/K
  Gain1 : Gain  Gain=T
  Sum : Sum  Inputs=|++
  Out1 : Outport
  wires:
  Gain/1 -> Gain1/1, Sum/1
  Sum/1 -> Out1/1
  Derivative/1 -> Sum/2
  Gain1/1 -> Derivative/1
  y+n/1 -> Gain/1

== system obs_com_filtro_2014/Dist_Observer3/G^{-1} ==
  y+n : Inport
  Derivative : Derivative  CoefficientInTFapproximation=1e-6
  Gain : Gain  Gain=1/K
  Gain1 : Gain  Gain=T
  Sum : Sum  Inputs=|++
  Out1 : Outport
  wires:
  Gain/1 -> Gain1/1, Sum/1
  Sum/1 -> Out1/1
  Derivative/1 -> Sum/2
  Gain1/1 -> Derivative/1
  y+n/1 -> Gain/1

== system obs_com_filtro_2014/Dist_Observer4/G^{-1} ==
  y+n : Inport
  Derivative : Derivative  CoefficientInTFapproximation=1e-6
  Gain : Gain  Gain=1/K
  Gain1 : Gain  Gain=T
  Sum : Sum  Inputs=|++
  Out1 : Outport
  wires:
  Gain/1 -> Gain1/1, Sum/1
  Sum/1 -> Out1/1
  Derivative/1 -> Sum/2
  Gain1/1 -> Derivative/1
  y+n/1 -> Gain/1

== system obs_com_filtro_2014/Dist_Observer5/G^{-1} ==
  y+n : Inport
  Derivative : Derivative  CoefficientInTFapproximation=1e-6
  Gain : Gain  Gain=1/K
  Gain1 : Gain  Gain=T
  Sum : Sum  Inputs=|++
  Out1 : Outport
  wires:
  Gain/1 -> Gain1/1, Sum/1
  Sum/1 -> Out1/1
  Derivative/1 -> Sum/2
  Gain1/1 -> Derivative/1
  y+n/1 -> Gain/1

== system obs_com_filtro_2014/Dist_Observer6/G^{-1} ==
  y+n : Inport
  Derivative : Derivative  CoefficientInTFapproximation=1e-6
  Gain : Gain  Gain=1/K
  Gain1 : Gain  Gain=T
  Sum : Sum  Inputs=|++
  Out1 : Outport
  wires:
  Gain/1 -> Gain1/1, Sum/1
  Sum/1 -> Out1/1
  Derivative/1 -> Sum/2
  Gain1/1 -> Derivative/1
  y+n/1 -> Gain/1

== system obs_com_filtro_2014/Dist_Observer7/G^{-1} ==
  y+n : Inport
  Derivative : Derivative  CoefficientInTFapproximation=1e-6
  Gain : Gain  Gain=1/K
  Gain1 : Gain  Gain=T
  Sum : Sum  Inputs=|++
  Out1 : Outport
  wires:
  Gain/1 -> Gain1/1, Sum/1
  Sum/1 -> Out1/1
  Derivative/1 -> Sum/2
  Gain1/1 -> Derivative/1
  y+n/1 -> Gain/1

== system obs_com_filtro_2014/Dist_Observer8/G^{-1} ==
  y+n : Inport
  Derivative : Derivative  CoefficientInTFapproximation=1e-6
  Gain : Gain  Gain=1/K
  Gain1 : Gain  Gain=T
  Sum : Sum  Inputs=|++
  Out1 : Outport
  wires:
  Gain/1 -> Gain1/1, Sum/1
  Sum/1 -> Out1/1
  Derivative/1 -> Sum/2
  Gain1/1 -> Derivative/1
  y+n/1 -> Gain/1

== system obs_com_filtro_2014/Dist_Observer9/G^{-1} ==
  y+n : Inport
  Derivative : Derivative  CoefficientInTFapproximation=1e-6
  Gain : Gain  Gain=1/K
  Gain1 : Gain  Gain=T
  Sum : Sum  Inputs=|++
  Out1 : Outport
  wires:
  Gain/1 -> Gain1/1, Sum/1
  Sum/1 -> Out1/1
  Derivative/1 -> Sum/2
  Gain1/1 -> Derivative/1
  y+n/1 -> Gain/1

== matlab function obs_com_filtro_2014/Statistic Filter2 ==
  settings: updateMethod=DISCRETE
  data: u input; saida_filtro output; std_dev parameter; alpha output
%Autor: Lucas Moura Gomes
%Filtro estatístico.

function [saida_filtro, alpha]  = filtroPID( u, std_dev)
    persistent x_ant;
    persistent alpha_orig;
    
    if isempty(x_ant)
        x_ant = 0;
        Ts = 0.01; %sampling time
        tf = 2; %continuous time cte.
        alpha_orig = 1 - exp(-1/tf * Ts); %c2d filter
    end
    
    alpha = erf(abs(x_ant - u)/(sqrt(2)*2*std_dev));
    
    if alpha > 1
        alpha = 1;
    end
    
    %up = 1.1; %upper bound 10%
    %alpha = alpha * alpha_orig * up;
    
    saida_filtro = (1-alpha)*x_ant + alpha*u;
    
    x_ant = saida_filtro;
end

%Autor: Lucas Moura Gomes
%Filtro estatístico.
% 
% function [saida_filtro, alpha] = filtroPID( u, erro_tipico_medicao, Tf  )
% 	
%     persistent x_ant;
%     
%     if isempty(x_ant)
%         x_ant = 0;
%     end
%     
%     Tf = Tf/1.5;
%     a_Tf = 1 - exp(-1/Tf * 5);
%     
%     alpha = erf(abs(x_ant - u)/(sqrt(2)*2*erro_tipico_medicao));
%     
%     if alpha > 1 
%         alpha = 1;
%     end;
%     
%     saida_filtro = (1-alpha)*x_ant + alpha*u;
% 
%     x_ant = saida_filtro;
%         
% 
%     saida_filtro = x_ant;
% 
%     
% end

== matlab function obs_com_filtro_2014/Dist_Observer1/MATLAB Function ==
  settings: updateMethod=DISCRETE
  data: u input; saida_filtro output; std_dev parameter; alpha output
%Autor: Lucas Moura Gomes
%Filtro estatístico.

function [saida_filtro, alpha]  = filtroPID( u, std_dev)
    persistent x_ant;
    persistent alpha_orig;
    
    if isempty(x_ant)
        x_ant = 0;
        alpha_orig = 1 - exp(-1/2 * 0.01);
    end;
    
    alpha = erf(abs(x_ant - u)/(sqrt(2)*2*std_dev));
    
    if alpha > 1
        alpha = 1;
    end;
    
    alpha = alpha * alpha_orig * 1.1;
    
    saida_filtro = (1-alpha)*x_ant + alpha*u;
    
    x_ant = saida_filtro;
end

== matlab function obs_com_filtro_2014/Statistic Filter5 ==
  settings: updateMethod=DISCRETE
  data: u input; saida_filtro output; std_dev parameter; alpha output
%Autor: Lucas Moura Gomes
%Filtro estatístico.

function [saida_filtro, alpha]  = filtroPID( u, std_dev)
    persistent x_ant;
    persistent alpha_orig;
    
    if isempty(x_ant)
        x_ant = 0;
        Ts = 0.01; %sampling time
        tf = 2; %continuous time cte.
        alpha_orig = 1 - exp(-1/tf * Ts); %c2d filter
    end
    
    alpha = erf(abs(x_ant - u)/(sqrt(2)*2*std_dev));
    
    if alpha > 1
        alpha = 1;
    end
    
    %up = 1.1; %upper bound 10%
    %alpha = alpha * alpha_orig * up;
    
    saida_filtro = (1-alpha)*x_ant + alpha*u;
    
    x_ant = saida_filtro;
end

%Autor: Lucas Moura Gomes
%Filtro estatístico.
% 
% function [saida_filtro, alpha] = filtroPID( u, erro_tipico_medicao, Tf  )
% 	
%     persistent x_ant;
%     
%     if isempty(x_ant)
%         x_ant = 0;
%     end
%     
%     Tf = Tf/1.5;
%     a_Tf = 1 - exp(-1/Tf * 5);
%     
%     alpha = erf(abs(x_ant - u)/(sqrt(2)*2*erro_tipico_medicao));
%     
%     if alpha > 1 
%         alpha = 1;
%     end;
%     
%     saida_filtro = (1-alpha)*x_ant + alpha*u;
% 
%     x_ant = saida_filtro;
%         
% 
%     saida_filtro = x_ant;
% 
%     
% end

== matlab function obs_com_filtro_2014/Dist_Observer12/Statistic Filter2 ==
  settings: updateMethod=DISCRETE
  data: u1 input; u2 input; saida_filtro1 output; saida_filtro2 output; std_dev parameter; alpha output; alpha_max parameter
%Autor: Lucas Moura Gomes
%Filtro estatístico.

function [saida_filtro1, saida_filtro2, alpha]  = filtroPID( u1, u2, std_dev, alpha_max)
    persistent x_ant1;
    persistent x_ant2;
    persistent alpha_orig;
    
    if isempty(x_ant1)
        x_ant1 = 0;
        Ts = 0.01; %sampling time
        tf = 2; %continuous time cte.
        alpha_orig = 1 - exp(-1/tf * Ts); %c2d filter
    end
    
    if isempty(x_ant2)
        x_ant2 = 0;
        Ts = 0.01; %sampling time
        tf = 2; %continuous time cte.
        alpha_orig = 1 - exp(-1/tf * Ts); %c2d filter
    end
    
    alpha = erf(abs(x_ant1 - u1)/(sqrt(2)*2*std_dev));
    
    if alpha > alpha_max
        alpha = alpha_max;
    end
    
    %up = 1.1; %upper bound 10%
    %alpha = alpha * alpha_orig * up;
    
    saida_filtro1 = (1-alpha)*x_ant1 + alpha*u1;
    saida_filtro2 = (1-alpha)*x_ant2 + alpha*u2;
    
    x_ant1 = saida_filtro1;
    x_ant2 = saida_filtro2;
end

%Autor: Lucas Moura Gomes
%Filtro estatístico.
% 
% function [saida_filtro, alpha] = filtroPID( u, erro_tipico_medicao, Tf  )
% 	
%     persistent x_ant1;
%     
%     if isempty(x_ant1)
%         x_ant1 = 0;
%     end
%     
%     Tf = Tf/1.5;
%     a_Tf = 1 - exp(-1/Tf * 5);
%     
%     alpha = erf(abs(x_ant1 - u)/(sqrt(2)*2*erro_tipico_medicao));
%     
%     if alpha > 1 
%         alpha = 1;
%     end;
%     
%     saida_filtro = (1-alpha)*x_ant1 + alpha*u;
% 
%     x_ant1 = saida_filtro;
%         
% 
%     saida_filtro = x_ant1;
% 
%     
% end

== matlab function obs_com_filtro_2014/Statistic Filter3 ==
  settings: updateMethod=DISCRETE
  data: u input; saida_filtro output; std_dev parameter; alpha output
%Autor: Lucas Moura Gomes
%Filtro estatístico.

function [saida_filtro, alpha]  = filtroPID( u, std_dev)
    persistent x_ant;
    persistent alpha_orig;
    
    if isempty(x_ant)
        x_ant = 0;
        Ts = 0.01; %sampling time
        tf = 2; %continuous time cte.
        alpha_orig = 1 - exp(-1/tf * Ts); %c2d filter
    end
    
    alpha = erf(abs(x_ant - u)/(sqrt(2)*2*std_dev));
    
    if alpha > 1
        alpha = 1;
    end
    
    %up = 1.1; %upper bound 10%
    %alpha = alpha * alpha_orig * up;
    
    saida_filtro = (1-alpha)*x_ant + alpha*u;
    
    x_ant = saida_filtro;
end

%Autor: Lucas Moura Gomes
%Filtro estatístico.
% 
% function [saida_filtro, alpha] = filtroPID( u, erro_tipico_medicao, Tf  )
% 	
%     persistent x_ant;
%     
%     if isempty(x_ant)
%         x_ant = 0;
%     end
%     
%     Tf = Tf/1.5;
%     a_Tf = 1 - exp(-1/Tf * 5);
%     
%     alpha = erf(abs(x_ant - u)/(sqrt(2)*2*erro_tipico_medicao));
%     
%     if alpha > 1 
%         alpha = 1;
%     end;
%     
%     saida_filtro = (1-alpha)*x_ant + alpha*u;
% 
%     x_ant = saida_filtro;
%         
% 
%     saida_filtro = x_ant;
% 
%     
% end

== matlab function obs_com_filtro_2014/Dist_Observer8/Statistic Filter3 ==
  settings: updateMethod=DISCRETE
  data: u input; saida_filtro output; std_dev parameter; alpha output
%Autor: Lucas Moura Gomes
%Filtro estatístico.

function [saida_filtro, alpha]  = filtroPID( u, std_dev)
    persistent x_ant;
    persistent alpha_orig;
    
    if isempty(x_ant)
        x_ant = 0;
        Ts = 0.01; %sampling time
        tf = 2; %continuous time cte.
        alpha_orig = 1 - exp(-1/tf * Ts); %c2d filter
    end
    
    alpha = erf(abs(x_ant - u)/(sqrt(2)*2*std_dev));
    
    if alpha > 1
        alpha = 1;
    end
    
    %up = 1.1; %upper bound 10%
    %alpha = alpha * alpha_orig * up;
    
    saida_filtro = (1-alpha)*x_ant + alpha*u;
    
    x_ant = saida_filtro;
end

%Autor: Lucas Moura Gomes
%Filtro estatístico.
% 
% function [saida_filtro, alpha] = filtroPID( u, erro_tipico_medicao, Tf  )
% 	
%     persistent x_ant;
%     
%     if isempty(x_ant)
%         x_ant = 0;
%     end
%     
%     Tf = Tf/1.5;
%     a_Tf = 1 - exp(-1/Tf * 5);
%     
%     alpha = erf(abs(x_ant - u)/(sqrt(2)*2*erro_tipico_medicao));
%     
%     if alpha > 1 
%         alpha = 1;
%     end;
%     
%     saida_filtro = (1-alpha)*x_ant + alpha*u;
% 
%     x_ant = saida_filtro;
%         
% 
%     saida_filtro = x_ant;
% 
%     
% end

== matlab function obs_com_filtro_2014/Dist_Observer5/Statistic Filter ==
  settings: updateMethod=DISCRETE
  data: u input; saida_filtro output; std_dev parameter; alpha output
%Autor: Lucas Moura Gomes
%Filtro estatístico.

function [saida_filtro, alpha]  = filtroPID( u, std_dev)
    persistent x_ant;
    persistent alpha_orig;
    
    if isempty(x_ant)
        x_ant = 0;
        Ts = 0.01; %sampling time
        tf = 2; %continuous time cte.
        alpha_orig = 1 - exp(-1/tf * Ts); %c2d filter
    end
    
    alpha = erf(abs(x_ant - u)/(sqrt(2)*2*std_dev));
    
    if alpha > 1
        alpha = 1;
    end
    
    %up = 1.1; %upper bound 10%
    %alpha = alpha * alpha_orig * up;
    
    saida_filtro = (1-alpha)*x_ant + alpha*u;
    
    x_ant = saida_filtro;
end

%Autor: Lucas Moura Gomes
%Filtro estatístico.
% 
% function [saida_filtro, alpha] = filtroPID( u, erro_tipico_medicao, Tf  )
% 	
%     persistent x_ant;
%     
%     if isempty(x_ant)
%         x_ant = 0;
%     end
%     
%     Tf = Tf/1.5;
%     a_Tf = 1 - exp(-1/Tf * 5);
%     
%     alpha = erf(abs(x_ant - u)/(sqrt(2)*2*erro_tipico_medicao));
%     
%     if alpha > 1 
%         alpha = 1;
%     end;
%     
%     saida_filtro = (1-alpha)*x_ant + alpha*u;
% 
%     x_ant = saida_filtro;
%         
% 
%     saida_filtro = x_ant;
% 
%     
% end

== matlab function obs_com_filtro_2014/Dist_Observer7/Statistic Filter ==
  settings: updateMethod=DISCRETE
  data: u input; saida_filtro output; std_dev parameter; alpha output
%Autor: Lucas Moura Gomes
%Filtro estatístico.

function [saida_filtro, alpha]  = filtroPID( u, std_dev)
    persistent x_ant;
    persistent alpha_orig;
    
    if isempty(x_ant)
        x_ant = 0;
        Ts = 0.01; %sampling time
        tf = 2; %continuous time cte.
        alpha_orig = 1 - exp(-1/tf * Ts); %c2d filter
    end
    
    alpha = erf(abs(x_ant - u)/(sqrt(2)*2*std_dev));
    
    if alpha > 1
        alpha = 1;
    end
    
    %up = 1.1; %upper bound 10%
    %alpha = alpha * alpha_orig * up;
    
    saida_filtro = (1-alpha)*x_ant + alpha*u;
    
    x_ant = saida_filtro;
end

%Autor: Lucas Moura Gomes
%Filtro estatístico.
% 
% function [saida_filtro, alpha] = filtroPID( u, erro_tipico_medicao, Tf  )
% 	
%     persistent x_ant;
%     
%     if isempty(x_ant)
%         x_ant = 0;
%     end
%     
%     Tf = Tf/1.5;
%     a_Tf = 1 - exp(-1/Tf * 5);
%     
%     alpha = erf(abs(x_ant - u)/(sqrt(2)*2*erro_tipico_medicao));
%     
%     if alpha > 1 
%         alpha = 1;
%     end;
%     
%     saida_filtro = (1-alpha)*x_ant + alpha*u;
% 
%     x_ant = saida_filtro;
%         
% 
%     saida_filtro = x_ant;
% 
%     
% end

== matlab function obs_com_filtro_2014/Dist_Observer8/Statistic Filter1111 ==
  settings: updateMethod=DISCRETE
  data: u input; saida_filtro output; std_dev parameter; alpha output
%Autor: Lucas Moura Gomes
%Filtro estatístico.

function [saida_filtro, alpha]  = filtroPID( u, std_dev)
    persistent x_ant;
    persistent alpha_orig;
    
    if isempty(x_ant)
        x_ant = 0;
        Ts = 0.01; %sampling time
        tf = 2; %continuous time cte.
        alpha_orig = 1 - exp(-1/tf * Ts); %c2d filter
    end
    
    alpha = erf(abs(x_ant - u)/(sqrt(2)*2*std_dev));
    
    if alpha > 1
        alpha = 1;
    end
    
    %up = 1.1; %upper bound 10%
    %alpha = alpha * alpha_orig * up;
    
    saida_filtro = (1-alpha)*x_ant + alpha*u;
    
    x_ant = saida_filtro;
end

%Autor: Lucas Moura Gomes
%Filtro estatístico.
% 
% function [saida_filtro, alpha] = filtroPID( u, erro_tipico_medicao, Tf  )
% 	
%     persistent x_ant;
%     
%     if isempty(x_ant)
%         x_ant = 0;
%     end
%     
%     Tf = Tf/1.5;
%     a_Tf = 1 - exp(-1/Tf * 5);
%     
%     alpha = erf(abs(x_ant - u)/(sqrt(2)*2*erro_tipico_medicao));
%     
%     if alpha > 1 
%         alpha = 1;
%     end;
%     
%     saida_filtro = (1-alpha)*x_ant + alpha*u;
% 
%     x_ant = saida_filtro;
%         
% 
%     saida_filtro = x_ant;
% 
%     
% end

== matlab function obs_com_filtro_2014/Dist_Observer10/Statistic Filter ==
  settings: updateMethod=DISCRETE
  data: u input; saida_filtro output; std_dev parameter; alpha output
%Autor: Lucas Moura Gomes
%Filtro estatístico.

function [saida_filtro, alpha]  = filtroPID( u, std_dev)
    persistent x_ant;
    persistent alpha_orig;
    
    if isempty(x_ant)
        x_ant = 0;
        Ts = 0.01; %sampling time
        tf = 2; %continuous time cte.
        alpha_orig = 1 - exp(-1/tf * Ts); %c2d filter
    end
    
    alpha = erf(abs(x_ant - u)/(sqrt(2)*2*std_dev));
    
    if alpha > 1
        alpha = 1;
    end
    
    %up = 1.1; %upper bound 10%
    %alpha = alpha * alpha_orig * up;
    
    saida_filtro = (1-alpha)*x_ant + alpha*u;
    
    x_ant = saida_filtro;
end

%Autor: Lucas Moura Gomes
%Filtro estatístico.
% 
% function [saida_filtro, alpha] = filtroPID( u, erro_tipico_medicao, Tf  )
% 	
%     persistent x_ant;
%     
%     if isempty(x_ant)
%         x_ant = 0;
%     end
%     
%     Tf = Tf/1.5;
%     a_Tf = 1 - exp(-1/Tf * 5);
%     
%     alpha = erf(abs(x_ant - u)/(sqrt(2)*2*erro_tipico_medicao));
%     
%     if alpha > 1 
%         alpha = 1;
%     end;
%     
%     saida_filtro = (1-alpha)*x_ant + alpha*u;
% 
%     x_ant = saida_filtro;
%         
% 
%     saida_filtro = x_ant;
% 
%     
% end

== matlab function obs_com_filtro_2014/Dist_Observer9/Statistic Filter ==
  settings: updateMethod=DISCRETE
  data: u input; saida_filtro output; std_dev parameter; alpha output
%Autor: Lucas Moura Gomes
%Filtro estatístico.

function [saida_filtro, alpha]  = filtroPID( u, std_dev)
    persistent x_ant;
    persistent alpha_orig;
    
    if isempty(x_ant)
        x_ant = 0;
        Ts = 0.01; %sampling time
        tf = 2; %continuous time cte.
        alpha_orig = 1 - exp(-1/tf * Ts); %c2d filter
    end
    
    alpha = erf(abs(x_ant - u)/(sqrt(2)*2*std_dev));
    
    if alpha > 1
        alpha = 1;
    end
    
    %up = 1.1; %upper bound 10%
    %alpha = alpha * alpha_orig * up;
    
    saida_filtro = (1-alpha)*x_ant + alpha*u;
    
    x_ant = saida_filtro;
end

%Autor: Lucas Moura Gomes
%Filtro estatístico.
% 
% function [saida_filtro, alpha] = filtroPID( u, erro_tipico_medicao, Tf  )
% 	
%     persistent x_ant;
%     
%     if isempty(x_ant)
%         x_ant = 0;
%     end
%     
%     Tf = Tf/1.5;
%     a_Tf = 1 - exp(-1/Tf * 5);
%     
%     alpha = erf(abs(x_ant - u)/(sqrt(2)*2*erro_tipico_medicao));
%     
%     if alpha > 1 
%         alpha = 1;
%     end;
%     
%     saida_filtro = (1-alpha)*x_ant + alpha*u;
% 
%     x_ant = saida_filtro;
%         
% 
%     saida_filtro = x_ant;
% 
%     
% end

== matlab function obs_com_filtro_2014/Statistic Filter4 ==
  settings: updateMethod=DISCRETE
  data: u input; saida_filtro output; std_dev parameter; alpha output
%Autor: Lucas Moura Gomes
%Filtro estatístico.

function [saida_filtro, alpha]  = filtroPID( u, std_dev)
    persistent x_ant;
    persistent alpha_orig;
    
    if isempty(x_ant)
        x_ant = 0;
        Ts = 0.01; %sampling time
        tf = 2; %continuous time cte.
        alpha_orig = 1 - exp(-1/tf * Ts); %c2d filter
    end
    
    alpha = erf(abs(x_ant - u)/(sqrt(2)*2*std_dev));
    
    if alpha > 1
        alpha = 1;
    end
    
    %up = 1.1; %upper bound 10%
    %alpha = alpha * alpha_orig * up;
    
    saida_filtro = (1-alpha)*x_ant + alpha*u;
    
    x_ant = saida_filtro;
end

%Autor: Lucas Moura Gomes
%Filtro estatístico.
% 
% function [saida_filtro, alpha] = filtroPID( u, erro_tipico_medicao, Tf  )
% 	
%     persistent x_ant;
%     
%     if isempty(x_ant)
%         x_ant = 0;
%     end
%     
%     Tf = Tf/1.5;
%     a_Tf = 1 - exp(-1/Tf * 5);
%     
%     alpha = erf(abs(x_ant - u)/(sqrt(2)*2*erro_tipico_medicao));
%     
%     if alpha > 1 
%         alpha = 1;
%     end;
%     
%     saida_filtro = (1-alpha)*x_ant + alpha*u;
% 
%     x_ant = saida_filtro;
%         
% 
%     saida_filtro = x_ant;
% 
%     
% end

== matlab function obs_com_filtro_2014/Statistic Filter6 ==
  settings: updateMethod=DISCRETE
  data: u input; saida_filtro output; std_dev parameter; alpha output
%Autor: Lucas Moura Gomes
%Filtro estatístico.

function [saida_filtro, alpha]  = filtroPID( u, std_dev)
    persistent x_ant;
    persistent alpha_orig;
    
    if isempty(x_ant)
        x_ant = 0;
        Ts = 0.01; %sampling time
        tf = 2; %continuous time cte.
        alpha_orig = 1 - exp(-1/tf * Ts); %c2d filter
    end
    
    alpha = erf(abs(x_ant - u)/(sqrt(2)*2*std_dev));
    
    if alpha > 1
        alpha = 1;
    end
    
    %up = 1.1; %upper bound 10%
    %alpha = alpha * alpha_orig * up;
    
    saida_filtro = (1-alpha)*x_ant + alpha*u;
    
    x_ant = saida_filtro;
end

%Autor: Lucas Moura Gomes
%Filtro estatístico.
% 
% function [saida_filtro, alpha] = filtroPID( u, erro_tipico_medicao, Tf  )
% 	
%     persistent x_ant;
%     
%     if isempty(x_ant)
%         x_ant = 0;
%     end
%     
%     Tf = Tf/1.5;
%     a_Tf = 1 - exp(-1/Tf * 5);
%     
%     alpha = erf(abs(x_ant - u)/(sqrt(2)*2*erro_tipico_medicao));
%     
%     if alpha > 1 
%         alpha = 1;
%     end;
%     
%     saida_filtro = (1-alpha)*x_ant + alpha*u;
% 
%     x_ant = saida_filtro;
%         
% 
%     saida_filtro = x_ant;
% 
%     
% end

== matlab function obs_com_filtro_2014/Statistic Filter1 ==
  settings: updateMethod=DISCRETE
  data: u input; saida_filtro output; std_dev parameter; alpha output
%Autor: Lucas Moura Gomes
%Filtro estatístico.

function [saida_filtro, alpha]  = filtroPID( u, std_dev)
    persistent x_ant;
    persistent alpha_orig;
    
    if isempty(x_ant)
        x_ant = 0;
        Ts = 0.01; %sampling time
        tf = 2; %continuous time cte.
        alpha_orig = 1 - exp(-1/tf * Ts); %c2d filter
    end
    
    alpha = erf(abs(x_ant - u)/(sqrt(2)*2*std_dev));
    
    if alpha > 1
        alpha = 1;
    end
    
    %up = 1.1; %upper bound 10%
    %alpha = alpha * alpha_orig * up;
    
    saida_filtro = (1-alpha)*x_ant + alpha*u;
    
    x_ant = saida_filtro;
end

%Autor: Lucas Moura Gomes
%Filtro estatístico.
% 
% function [saida_filtro, alpha] = filtroPID( u, erro_tipico_medicao, Tf  )
% 	
%     persistent x_ant;
%     
%     if isempty(x_ant)
%         x_ant = 0;
%     end
%     
%     Tf = Tf/1.5;
%     a_Tf = 1 - exp(-1/Tf * 5);
%     
%     alpha = erf(abs(x_ant - u)/(sqrt(2)*2*erro_tipico_medicao));
%     
%     if alpha > 1 
%         alpha = 1;
%     end;
%     
%     saida_filtro = (1-alpha)*x_ant + alpha*u;
% 
%     x_ant = saida_filtro;
%         
% 
%     saida_filtro = x_ant;
% 
%     
% end
